simulink model "bernuli1"  (Simulink 7.9)
settings: Solver=ode45  StartTime=-10.0  StopTime=100.0  RelTol=1e-3
libraries: simulink x2
settings Model: Creator=Mihail  LastModifiedBy=Mihail

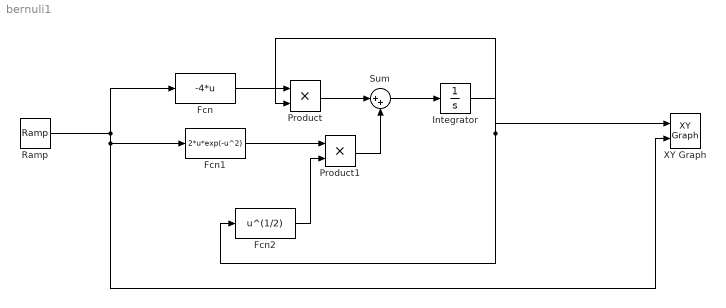
== system bernuli1 ==
  Fcn : Fcn  Expr=-4*u
  Fcn1 : Fcn  Expr=2*u*exp(-u^2)
  Fcn2 : Fcn  Expr=u^(1/2)
  Integrator : Integrator  InitialCondition=1
  Product : Product  RndMeth=Zero
  Product1 : Product  RndMeth=Zero
  Ramp : simulink/Sources/Ramp  slope=1  start=0  X0=1
  Sum : Sum  Inputs=|++
  XY Graph : simulink/Sinks/XY Graph  xmin=-1  xmax=1  ymin=0  ymax=5  st=-1
  wires:
  Integrator/1 -> Product/2, Fcn2/1, XY Graph/1
  Product/1 -> Sum/1
  Sum/1 -> Integrator/1
  Fcn/1 -> Product/1
  Ramp/1 -> Fcn1/1, Fcn/1, XY Graph/2
  Fcn1/1 -> Product1/1
  Product1/1 -> Sum/2
  Fcn2/1 -> Product1/2
